simulink model "ramps_as_inputs"  (R2015b)
settings: Solver=VariableStepAuto  StartTime=0.0  StopTime=200  RelTol=1e-3
libraries: simulink x4, fuzblock x1
settings Model: Creator=giorgos  LastModifiedBy=giorgos

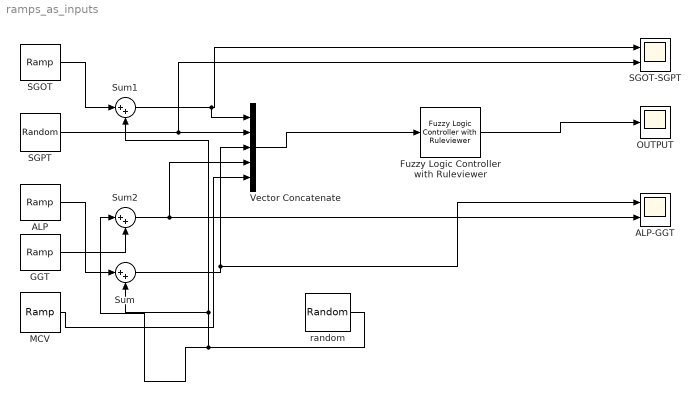
== system ramps_as_inputs ==
  ALP : simulink/Sources/Ramp  slope=0.8  start=0  X0=30
  ALP-GGT : Scope  NumInputPorts=2
  Fuzzy Logic Controller with Ruleviewer : fuzblock/Fuzzy Logic  Controller  with Ruleviewer  fismatrix=a  Ts=5
  GGT : simulink/Sources/Ramp  slope=0.4  start=0  X0=5
  "MCV " : simulink/Sources/Ramp  slope=0.1  start=0  X0=75
  OUTPUT : Scope
  SGOT : simulink/Sources/Ramp  slope=0.3  start=0  X0=7
  SGOT-SGPT : Scope  NumInputPorts=2
  SGPT : UniformRandomNumber  Minimum=10  Maximum=30  Seed=1  SampleTime=5
  Sum : Sum  Inputs=|++
  Sum1 : Sum  Inputs=|++
  Sum2 : Sum  Inputs=|++
  Vector Concatenate : Concatenate  NumInputs=5
  random : UniformRandomNumber  Minimum=-3  Maximum=5  Seed=1  SampleTime=5
  wires:
  "MCV "/1 -> Vector Concatenate/5
  Vector Concatenate/1 -> Fuzzy Logic Controller with Ruleviewer/1
  Fuzzy Logic Controller with Ruleviewer/1 -> OUTPUT/1
  SGPT/1 -> SGOT-SGPT/2, Vector Concatenate/2
  random/1 -> Sum2/1, Sum/2, Sum1/2
  ALP/1 -> Sum/1
  Sum/1 -> ALP-GGT/1, Vector Concatenate/3
  SGOT/1 -> Sum1/1
  Sum1/1 -> Vector Concatenate/1, SGOT-SGPT/1
  GGT/1 -> Sum2/2
  Sum2/1 -> ALP-GGT/2, Vector Concatenate/4
